simulink model "Avoid_vat_can_1xe"  (R2021b)
settings: Solver=FixedStepAuto  StartTime=0.0  StopTime=120  FixedStep=0.01  RelTol=1e-3
model workspace (MAT data in the model file):
  Data_robot = 1
values from neighbouring files (symbols this model uses):
  G_target = [5.8;8.0]    [parameter.m]
  Position_first_vehicle = [Set_first(1);Set_first(2);deg2rad(19.5)]    [parameter.m]
  Q_can = [4.4;7.2]    [parameter.m]
settings Model: Creator=HL_1810  LastModifiedBy=HL_1810
settings DebuggingCC: UnderSpecifiedDimensionMsg=error

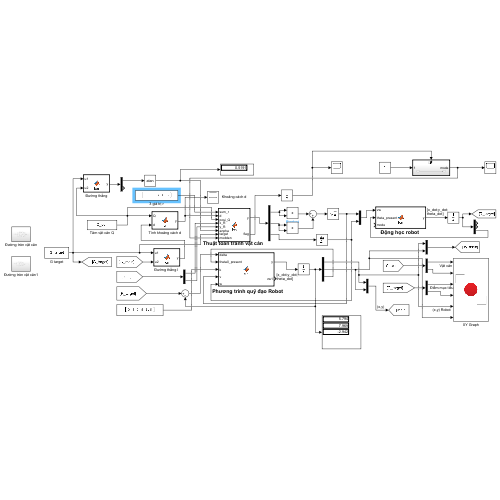
[thumbnail: Simulink's stored preview of the top-level diagram]
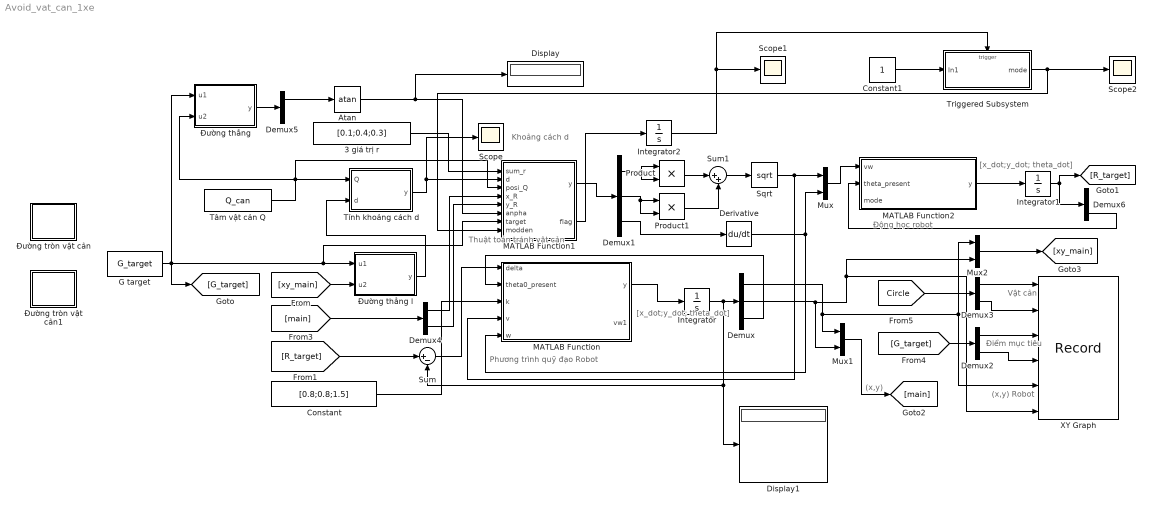
== system Avoid_vat_can_1xe ==
  note: Khoảng cách d
  note: (x,y) Robot
  note: Điểm mục tiêu
  note: Vật cản
  note: (x,y)
  note: [x_dot;y_dot;
      | theta_dot]
  note: Động học robot
  note: Thuật toán tránh vật cản
  note: Phương trình quỹ đạo Robot
  note: [x_dot;y_dot;
      | theta_dot]
  3 giá trị r : Constant  Value=[0.1;0.4;0.3]
  Atan : Trigonometry  Operator=atan
  Constant : Constant  Value=[0.8;0.8;1.5]
  Constant1 : Constant
  Demux : Demux  Outputs=3
  Demux1 : Demux  Outputs=3
  Demux{2..5} (4 alike) : Demux  Outputs=2
  Demux6 : Demux  Outputs=3
  Derivative : Derivative
  Display : Display
  Display1 : Display
  G target : Constant  Value=G_target
  Integrator : Integrator  InitialCondition=Position_first_vehicle
  Integrator1 : Integrator  InitialCondition=Position_first_vehicle
  Integrator2 : Integrator
  MATLAB Function : MATLAB Function  TreatAsAtomicUnit=on
  MATLAB Function1 : MATLAB Function  TreatAsAtomicUnit=on
  MATLAB Function2 : MATLAB Function  TreatAsAtomicUnit=on
  Mux : Mux  Inputs=2
  Mux1 : Mux  Inputs=2
  Mux2 : Mux  Inputs=2
  Product : Product
  Product1 : Product
  Scope : Scope
  Scope1 : Scope
  Scope2 : Scope
  Sqrt : Sqrt  SaturateOnIntegerOverflow=on
  Sum : Sum  Inputs=|+-
  Sum1 : Sum  Inputs=|++
  Triggered Subsystem : Subsystem  TreatAsAtomicUnit=on
  Tâm vật cản Q : Constant  Value=Q_can
  Tính khoảng cách d : MATLAB Function  TreatAsAtomicUnit=on
  XY Graph : Record  FileSettingsInternal="{\"entries\":[{\"content\":{\"excelSettings\":{\"content\":{},\"type\":\"Streamout.ExcelSettings\"}},\"type\":\"Streamout.FileSettingStorage\",\"uuid\":\"d028dad2-fe41-4f29-b7cf-11e89291ac11\"}],\"packageUris\":[\"http://schema.mathworks.com/mf0/streamout_blocks/R2020a\"],\"version\":\"1.0\"}"  Layout=[1 1]  SignalsInternal="{\"entries\":[{\"content\":{\"signals\":[{\"content\":{\"blockPath\":[\"Avoid_vat_can_1xe/XY Graph\"],\"channel\":[],\"dimensions\":[1],\"domain\":\"Avoid_vat_can_1xe/XY Graph\",\"lineColor\":\"#ff6929\",\"plots\":[1],\"port\":1,\"sid\":[\"\"],\"signalID\":232,\"signalName\":\"Demux3:1\"},\"type\":\"RecordBlkView.Signal\",\"uuid\":\"5252b280-9464-4429-a510-c86b50e29c90\"},{\"content\":{\"blockPath\":[\"Avoid_vat_can_1xe/XY Graph\"],\"channel\":[],\"dimensions\":[1],\"domain\":\"Avoid_vat_can_1xe/XY Graph\",\"lineColor\":\"#b746ff\",\"plots\":[1],\"port\":2,\"sid\":[\"\"],\"signalID\":236,\"signalName\":\"Demux3:2\"},\"type\":\"RecordBlkView.Signal\",\"uuid\":\"3d03e405-65f7-491b-9fcd-2c94ae8fbced\"},{\"content\":{\"blockPath\":[\"Avoid_vat_can_1xe/XY Graph\"],\"channel\":[],\"dimensions\":[1],\"domain\":\"Avoid_vat_can_1xe/XY Graph\",\"lineColor\":\"#64d413\",\"plots\":[1],\"port\":5,\"sid\":[\"\"],\"signalID\":240,\"signalName\":\"Demux:1\"},\"type\":\"RecordBlkView.Signal\",\"uuid\":\"be1e0271-cc7f-4b22-8700-58677786251a\"},{\"content\":{\"blockPath\":[\"Avoid_vat_can_1xe/XY Graph\"],\"channel\":[],\"dimensions\":[1],\"domain\":\"Avoid_vat_can_1xe/XY Graph\",\"lineColor\":\"#ff13a6\",\"plots\":[1],\"port\":6,\"sid\":[\"\"],\"signalID\":244,\"signalName\":\"Demux:2\"},\"type\":\"RecordBlkView.Signal\",\"uuid\":\"71d04cfa-f5db-4231-9a4a-18f1c7c31a28\"},{\"content\":{\"blockPath\":[\"Avoid_vat_can_1xe/XY Graph\"],\"channel\":[],\"dimensions\":[1],\"domain\":\"Avoid_vat_can_1xe/XY Graph\",\"lineColor\":\"#fe330a\",\"plots\":[1],\"port\":3,\"sid\":[\"\"],\"signalID\":248,\"signalName\":\"Demux2:1\"},\"type\":\"RecordBlkView.Signal\",\"uuid\":\"e42d958d-89b0-40d3-81a2-ec98c2b55a4d\"},{\"content\":{\"blockPath\":[\"Avoid_vat_can_1xe/XY Graph\"],\"channel\":[],\"dimensions\":[1],\"domain\":\"Avoid_vat_can_1xe/XY Graph\",\"lineColor\":\"#22b573\",\"plots\":[1],\"port\":4,\"sid\":[\"\"],\"signalID\":252,\"signalName\":\"Demux2:2\"},\"type\":\"RecordBlkView.Signal\",\"uuid\":\"f4eccc4a-794c-493c-b38d-a8020f4bd00a\"}]},\"type\":\"RecordBlkView.InputSignals\",\"uuid\":\"4d09d0e0-84fe-450c-8ad6-42e1c2b76c1f\"}],\"packageUris\":[\"http://schema.mathworks.com/mf0/streamout_blocks/R2020a\"],\"version\":\"1.0\"}"  VisualizationBindings="{\"xyplotplugin\":{\"info\":[{\"series\":[{\"bindingParametersList\":[{\"parameter\":\"X-Axis\",\"signalID\":232,\"signalName\":\"Demux3:1\"},{\"parameter\":\"Y-Axis\",\"signalID\":236,\"signalName\":\"Demux3:2\"}],\"seriesID\":42404},{\"bindingParametersList\":[{\"parameter\":\"X-Axis\",\"signalID\":240,\"signalName\":\"Demux:1\"},{\"parameter\":\"Y-Axis\",\"signalID\":244,\"signalName\":\"Demux:2\"}],\"seriesID\":45031},{\"bindingParametersList\":[{\"parameter\":\"X-Axis\",\"signalID\":248,\"signalName\":\"Demux2:1\"},{\"parameter\":\"Y-Axis\",\"signalID\":252,\"signalName\":\"Demux2:2\"}],\"seriesID\":38751}],\"subplotID\":1},{\"series\":[],\"subplotID\":2}]}}"  CompatibilityTag=XY
  Đường thẳng : MATLAB Function  TreatAsAtomicUnit=on
  "Đường thẳng l " : MATLAB Function  TreatAsAtomicUnit=on
  Đường tròn vật cản : Subsystem
  Đường tròn vật cản1 : Subsystem
  wires:
  Integrator/1 -> Demux/1, Display1/1, Sum/2
  MATLAB Function/1(y) -> Integrator/1
  Sum/1 -> MATLAB Function/1(delta)
  Constant/1 -> MATLAB Function/3(k)
  G target/1 -> [G_target], Đường thẳng/1(u1), MATLAB Function1/7(target), "Đường thẳng l "/1(u1)
  Tâm vật cản Q/1 -> Tính khoảng cách d/1(Q), Đường thẳng/2(u2), MATLAB Function1/3(posi_Q)
  "Đường thẳng l "/1(y) -> Tính khoảng cách d/2(d)
  Tính khoảng cách d/1(y) -> Scope/1, MATLAB Function1/2(d)
  3 giá trị r/1 -> MATLAB Function1/1(sum_r)
  MATLAB Function1/1(y) -> Demux1/1
  Demux1/1 -> Product/2, Product/1
  Demux1/2 -> Product1/2, Product1/1
  Demux1/3 -> Derivative/1
  Product/1 -> Sum1/1
  Product1/1 -> Sum1/2
  Sum1/1 -> Sqrt/1
  [Circle] -> Demux3/1
  Demux3/1 -> XY Graph/1
  Demux3/2 -> XY Graph/2
  Demux/1 -> XY Graph/5, Mux2/1, Mux1/1
  Demux/2 -> Mux1/2, XY Graph/6, Mux2/2
  [G_target] -> Demux2/1
  Demux2/1 -> XY Graph/3
  Demux2/2 -> XY Graph/4
  Sqrt/1 -> Mux/1, MATLAB Function/4(v)
  Derivative/1 -> MATLAB Function/5(w), Mux/2
  Mux/1 -> MATLAB Function2/1(vw)
  Demux4/1 -> MATLAB Function1/4(x_R)
  Demux4/2 -> MATLAB Function1/5(y_R)
  Mux1/1 -> [main]
  [main] -> Demux4/1
  Demux5/1 -> Atan/1
  Atan/1 -> Display/1, MATLAB Function1/6(anpha)
  MATLAB Function2/1(y) -> Integrator1/1
  Integrator1/1 -> Demux6/1, [R_target]
  Demux6/3 -> MATLAB Function2/2(theta_present)
  [R_target] -> Sum/1
  Đường thẳng/1(y) -> Demux5/1
  Mux2/1 -> [xy_main]
  [xy_main] -> "Đường thẳng l "/2(u2)
  Demux/3 -> MATLAB Function/2(theta0_present)
  Constant1/1 -> Triggered Subsystem/1(In1)
  Triggered Subsystem/1(mode) -> MATLAB Function1/8(modden), Scope2/1
  MATLAB Function1/2(flag) -> Integrator2/1
  Integrator2/1 -> Triggered Subsystem/Trigger, Scope1/1

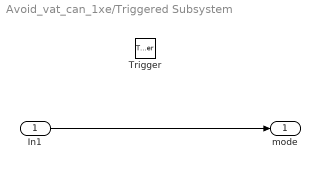
== system Avoid_vat_can_1xe/Triggered Subsystem ==
  In1 : Inport
  Trigger : TriggerPort  VariantControl=(inherit)
  mode : Outport
  wires:
  In1/1 -> mode/1

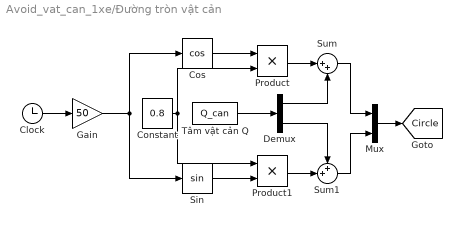
== system Avoid_vat_can_1xe/Đường tròn vật cản ==
  Clock : Clock
  Constant : Constant  Value=0.8
  Cos : Trigonometry  Operator=cos
  Demux : Demux  Outputs=2
  Gain : Gain  Gain=50
  Mux : Mux  Inputs=2
  Product : Product
  Product1 : Product
  Sin : Trigonometry
  Sum : Sum  Inputs=|++
  Sum1 : Sum  Inputs=++|
  Tâm vật cản Q : Constant  Value=Q_can
  tag scope: Circle=global
  wires:
  Product1/1 -> Sum1/2
  Constant/1 -> Product1/1, Product/2
  Product/1 -> Sum/1
  Sum/1 -> Mux/1
  Cos/1 -> Product/1
  Sum1/1 -> Mux/2
  Mux/1 -> [Circle]
  Clock/1 -> Gain/1
  Gain/1 -> Sin/1, Cos/1
  Sin/1 -> Product1/2
  Tâm vật cản Q/1 -> Demux/1
  Demux/1 -> Sum/2
  Demux/2 -> Sum1/1

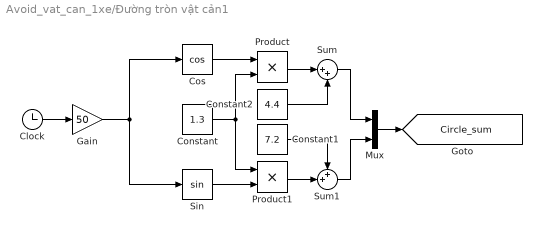
== system Avoid_vat_can_1xe/Đường tròn vật cản1 ==
  Clock : Clock
  Constant : Constant  Value=1.3
  Constant1 : Constant  Value=7.2
  Constant2 : Constant  Value=4.4
  Cos : Trigonometry  Operator=cos
  Gain : Gain  Gain=50
  Mux : Mux  Inputs=2
  Product : Product
  Product1 : Product
  Sin : Trigonometry
  Sum : Sum  Inputs=|++
  Sum1 : Sum  Inputs=++|
  tag scope: Circle_sum=global
  wires:
  Sin/1 -> Product1/2
  Gain/1 -> Cos/1, Sin/1
  Clock/1 -> Gain/1
  Constant1/1 -> Sum1/1
  Constant2/1 -> Sum/2
  Mux/1 -> [Circle_sum]
  Sum1/1 -> Mux/2
  Cos/1 -> Product/1
  Sum/1 -> Mux/1
  Product/1 -> Sum/1
  Constant/1 -> Product/2, Product1/1
  Product1/1 -> Sum1/2

== matlab function Avoid_vat_can_1xe/Đường thẳng l  ==
  data: u1 input; y output; u2 input
function y = fcn(u1,u2)
%#codegen
% Đường thẳng từ tâm Robot đến điểm mục tiêu
a=(u1(2)-u2(2))/(u1(1)-u2(1));
b=u1(2)-u1(1)*a;
u=[a;b];
y = u;

== matlab function Avoid_vat_can_1xe/MATLAB Function ==
  data: delta input; y output; theta0_present input; k input; v input; w input; vw1 output
function [y,vw1] = fcn(delta,theta0_present,k,v,w)
%#codegen
A=[cos(theta0_present)   sin(theta0_present) 0;
    -sin(theta0_present) cos(theta0_present) 0;
    0                    0                    1];
e=A*delta;
V_c=[v*cos(e(3))+k(1)*e(1);
    w+k(2)*v*e(2)+k(3)*v*sin(e(3))];

Matrix=[cos(theta0_present) 0;
        sin(theta0_present) 0;
        0                   1];
u=Matrix*V_c;
vw1=V_c;
y = u;

== matlab function Avoid_vat_can_1xe/Tính khoảng cách d ==
  data: Q input; y output; d input
function y = fcn(Q,d)
%#codegen
a=d(1);
b=-1;
c=d(2);
u=( Q(1)*a + b*Q(2) +c )/sqrt(a^2+b^2);
y = u;

== matlab function Avoid_vat_can_1xe/MATLAB Function1 ==
  data: sum_r input; y output; d input; posi_Q input; x_R input; y_R input; anpha input; target input; flag output; modden input
function [y,flag]= fcn(sum_r,d,posi_Q,x_R,y_R,anpha,target,modden)
%#codegen
rv=sum_r(1)+sum_r(2)+sum_r(3);



M=[cos(anpha) -sin(anpha) 0 posi_Q(1);
    sin(anpha) cos(anpha) 0 posi_Q(2);
    0 0 1 0;
    0 0 0 1];
N=[x_R;y_R;0;1];
Vitri=inv(M)*N;
dd=abs(1.697*x_R-y_R-1.842)/sqrt(1.697^2+1);
if ((d<rv) &&(dd>0.1))
    mode=0;
else
    mode=1;

end

if (modden==0)
        xr_dot=(d/abs(d))*Vitri(2)+Vitri(1)*(rv^2-Vitri(1)^2-Vitri(2)^2);
        yr_dot=-(d/abs(d))*Vitri(1)+Vitri(2)*(rv^2-Vitri(1)^2-Vitri(2)^2);
        theta_r=atan(yr_dot/xr_dot);
else
    if ((x_R-target(1))^2+(y_R-target(2))^2) > 0.001
            xr_dot = 0.04*cos(atan((y_R)-target(2))/((x_R)-target(1)));
            yr_dot = 0.04*sin(atan((y_R)-target(2))/((x_R)-target(1)));
            theta_r = atan((y_R)-target(2))/((x_R)-target(1));
        else 
            xr_dot = 0;
            yr_dot = 0;
            theta_r =0 ;
    end
end



u=[xr_dot;yr_dot;theta_r];

y = u;
flag=mode;

== matlab function Avoid_vat_can_1xe/MATLAB Function2 ==
  data: vw input; y output; theta_present input; mode input
function y = fcn(vw,theta_present,mode)
%#codegen
% if (mode==0)
%     vw1=[vw(1);vw(2)];
% else
%     vw1=[0.04;0];
% end
Matrix=[cos(theta_present) 0;
        sin(theta_present) 0;
        0                   1];
u=Matrix*vw;
y = u;

== matlab function Avoid_vat_can_1xe/Đường thẳng ==
  data: u1 input; y output; u2 input
function y = fcn(u1,u2)
%Đường thẳng từ mục tiêu đến tâm vật cản
a=(u1(2)-u2(2))/(u1(1)-u2(1)); %hệ số góc
b=u1(2)-u1(1)*a;
u=[a;b];
y = u;
